simulink model "wam_v_controller"  (R2017b)
settings: Solver=VariableStepAuto  StartTime=0.0  StopTime=10.0  RelTol=1e-3
libraries: robotlib x3
settings Model: Creator=masaya  LastModifiedBy=masaya

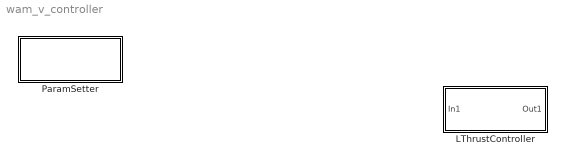
== system wam_v_controller ==
  LThrustController : Subsystem
  ParamSetter : Subsystem

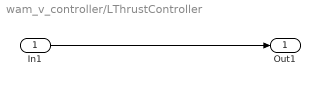
== system wam_v_controller/LThrustController ==
  In1 : Inport
  Out1 : Outport
  wires:
  In1/1 -> Out1/1

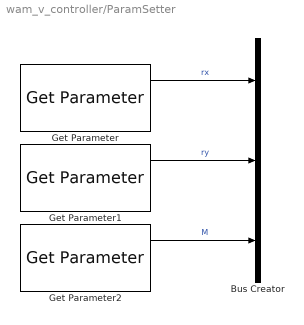
== system wam_v_controller/ParamSetter ==
  Bus Creator : BusCreator  Inputs=3
  Get Parameter : robotlib/Get Parameter  SourceLibraryInfo=This block requires Robotics System Toolbox  ParameterSource=Specify your own  ParameterName=/wam_v_controller/rx  ParameterType=double  ParameterMaxArrayLength=16  ParameterInitialValue=1.5  SampleTime=-1  ShowErrorCodeOutput=on  ModelName=wam_v_controller  BlockId=ParamGet_wam_v_controller_4
      settings: SourceProductName=Robotics System Toolbox  SourceProductBaseCode=RO
  Get Parameter1 : robotlib/Get Parameter  SourceLibraryInfo=This block requires Robotics System Toolbox  ParameterSource=Specify your own  ParameterName=/wam_v_controller/ry  ParameterType=double  ParameterMaxArrayLength=16  ParameterInitialValue=1.5  SampleTime=-1  ShowErrorCodeOutput=on  ModelName=wam_v_controller  BlockId=ParamGet_wam_v_controller_9
      settings: SourceProductName=Robotics System Toolbox  SourceProductBaseCode=RO
  Get Parameter2 : robotlib/Get Parameter  SourceLibraryInfo=This block requires Robotics System Toolbox  ParameterSource=Specify your own  ParameterName=/wam_v_controller/M  ParameterType=double  ParameterMaxArrayLength=16  ParameterInitialValue=250  SampleTime=-1  ShowErrorCodeOutput=on  ModelName=wam_v_controller  BlockId=ParamGet_wam_v_controller_11
      settings: SourceProductName=Robotics System Toolbox  SourceProductBaseCode=RO
  wires:
  Get Parameter/1 -> Bus Creator/1  "rx"
  Get Parameter1/1 -> Bus Creator/2  "ry"
  Get Parameter2/1 -> Bus Creator/3  "M"
